simulink model "scdspeed_ctrlloop"  (Simulink 7.6)
settings: Solver=ode45  StartTime=0  StopTime=15  MaxStep=0.01  RelTol=1e-3
libraries: simulink x1
settings Model: Creator=The MathWorks Inc.  BufferReuse=off
settings DataIOCC: ExternalInput=[0 0]  InitialState=xstr  LimitDataPoints=off  SaveFormat=StructureWithTime  SignalLoggingName=sigsout
settings OptimizationCC: InlineParams=on  InlineInvariantSignals=on  BufferReuse=off  InitFltsAndDblsToZero=on
settings DebuggingCC: AlgebraicLoopMsg=none  CheckExecutionContextPreStartOutputMsg=on  CheckExecutionContextRuntimeOutputMsg=on  SignalResolutionControl=TryResolveAllWithWarning  SolverPrmCheckMsg=none  MultiTaskDSMMsg=warning  StrictBusMsg=None
settings CodeAppCC: CustomSymbolStrFcn=$F$N$M

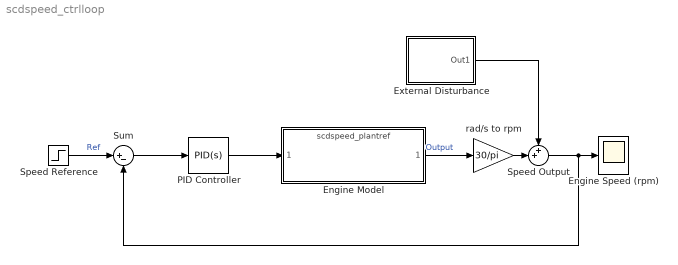
== system scdspeed_ctrlloop ==
  Engine Speed (rpm) : Scope
      settings: TickLabels=on  TimeRange=15  YMin=1500  YMax=3500  SaveName=N  DataFormat=Structure
  Engine Model : ModelReference  ModelNameDialog=scdspeed_plantref  SimulationMode=Accelerator  ModelReferenceVersion=1.33  CopyOfModelName=scdspeed_plantref
  External Disturbance : Subsystem
      settings: RTWMemSecFuncInitTerm=Default  RTWMemSecFuncExecute=Default  RTWMemSecDataConstants=Default  RTWMemSecDataInternal=Default  RTWMemSecDataParameters=Default
  PID Controller : simulink/Continuous/PID Controller  Tag=PID1  DialogController=pidpack.PIDConfig.pidDDGCreate  DialogControllerArgs=DataTag0  SystemSampleTime=-1  Controller=PID  TimeDomain=Continuous-time  SampleTime=1  IntegratorMethod=Forward Euler  FilterMethod=Forward Euler  Form=Parallel  P=0.0012191  I=0.0030038  D=0  N=100  InitialConditionSource=internal  InitialConditionForIntegrator=8.96  InitialConditionForFilter=0  ExternalReset=none  ZeroCross=off  LimitOutput=off  UpperSaturationLimit=inf  LowerSaturationLimit=-inf  LinearizeAsGain=off  AntiWindupMode=none  Kb=1  TrackingMode=off  Kt=1  PParamMin=[ ]  PParamMax=[ ]  IParamMin=[ ]  IParamMax=[ ]  DParamMin=[ ]  DParamMax=[ ]  NParamMin=[ ]  NParamMax=[ ]  KbParamMin=[ ]  KbParamMax=[ ]  KtParamMin=[ ]  KtParamMax=[ ]  POutMin=[ ]  POutMax=[ ]  IOutMin=[ ]  IOutMax=[ ]  DOutMin=[ ]  DOutMax=[ ]  NOutMin=[ ]  NOutMax=[ ]  KbOutMin=[ ]  KbOutMax=[ ]  KtOutMin=[ ]  KtOutMax=[ ]  IntegratorOutMin=[ ]  IntegratorOutMax=[ ]  FilterOutMin=[ ]  FilterOutMax=[ ]  SumOutMin=[ ]  SumOutMax=[ ]  SumI1OutMin=[ ]  SumI1OutMax=[ ]  SumI2OutMin=[ ]  SumI2OutMax=[ ]  SumI3OutMin=[ ]  SumI3OutMax=[ ]  SumDOutMin=[ ]  SumDOutMax=[ ]  SaturationOutMin=[ ]  SaturationOutMax=[ ]  IntegratorContinuousStateAttributes=''  IntegratorStateMustResolveToSignalObject=off  IntegratorRTWStateStorageClass=Auto  FilterContinuousStateAttributes=''  FilterStateMustResolveToSignalObject=off  FilterRTWStateStorageClass=Auto
  Speed Reference : Step  Time=2  Before=2000  After=3000  SampleTime=0
  Speed Output : Sum  Inputs=++|
  Sum : Sum  Inputs=|+-
  rad/s to rpm : Gain  Gain=30/pi  SaturateOnIntegerOverflow=on  OutDataTypeStr=Inherit: Same as input  ParamDataTypeStr=Inherit: Same as input
  wires:
  Sum/1 -> PID Controller/1
  Speed Reference/1 -> Sum/1  "Ref"
  PID Controller/1 -> Engine Model/1
  rad/s to rpm/1 -> Speed Output/2
  External Disturbance/1(Out1) -> Speed Output/1
  Engine Model/1 -> rad/s to rpm/1  "Output"
  Speed Output/1 -> Engine Speed (rpm)/1, Sum/2

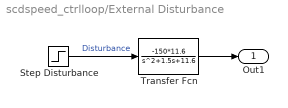
== system scdspeed_ctrlloop/External Disturbance ==
  Step Disturbance : Step  Time=10  SampleTime=0
  Transfer Fcn : TransferFcn  Numerator=-150*11.6  Denominator=[1 1.5 11.6]
  Out1 : Outport
  wires:
  Transfer Fcn/1 -> Out1/1
  Step Disturbance/1 -> Transfer Fcn/1  "Disturbance"
